simulink model "smlnk_hw4"  (R2019b)
settings: Solver=VariableStepAuto  StartTime=0.0  StopTime=15  RelTol=1e-3
undefined symbols (not defined in the file): C, m, sys, x0
settings Model: Creator=maximemeurisse  LastModifiedBy=maximemeurisse

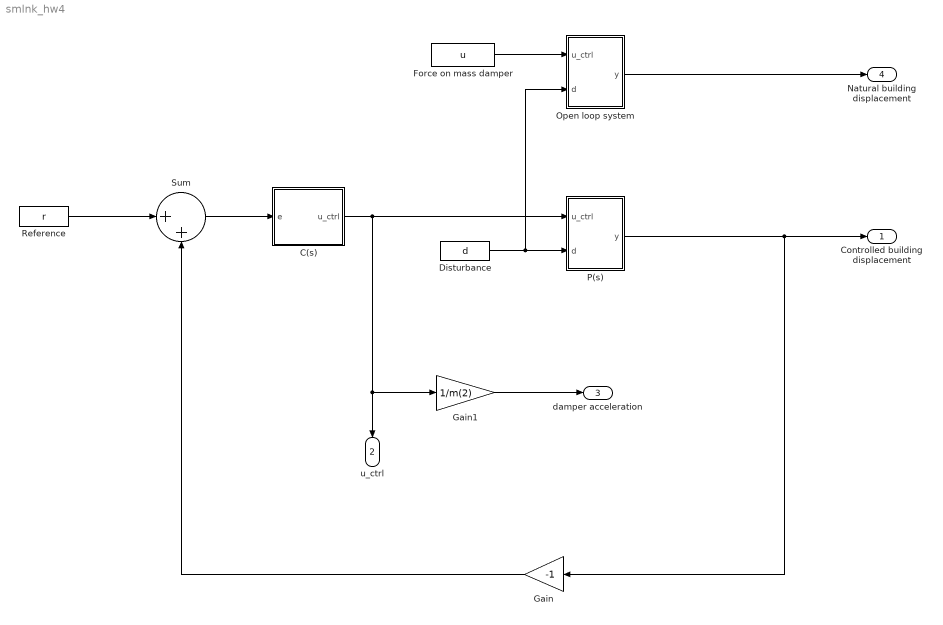
== system smlnk_hw4 ==
  C(s) : Subsystem
  Disturbance : FromWorkspace  VariableName=d  SampleTime=0
  Force on mass damper : FromWorkspace  VariableName=u  SampleTime=0
  Gain : Gain  Gain=-1
  Gain1 : Gain  Gain=1/m(2)
  Open loop system : Subsystem
  P(s) : Subsystem
  Reference : FromWorkspace  VariableName=r  SampleTime=0
  Sum : Sum  Inputs=|++
  Controlled building displacement : Outport
  u_ctrl : Outport  Port=2
  damper acceleration : Outport  Port=3
  Natural building displacement : Outport  Port=4
  wires:
  Gain/1 -> Sum/2
  Sum/1 -> C(s)/1(e)
  Reference/1 -> Sum/1
  Gain1/1 -> damper acceleration/1
  C(s)/1(u_ctrl) -> P(s)/1(u_ctrl), u_ctrl/1, Gain1/1
  P(s)/1(y) -> Gain/1, Controlled building displacement/1
  Disturbance/1 -> Open loop system/2(d), P(s)/2(d)
  Open loop system/1(y) -> Natural building displacement/1
  Force on mass damper/1 -> Open loop system/1(u_ctrl)

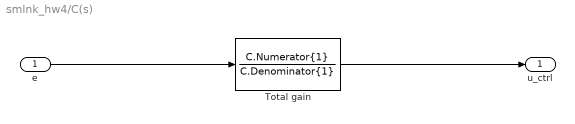
== system smlnk_hw4/C(s) ==
  e : Inport
  Total gain : TransferFcn  Numerator=C.Numerator{1}  Denominator=C.Denominator{1}
  u_ctrl : Outport
  wires:
  e/1 -> Total gain/1
  Total gain/1 -> u_ctrl/1

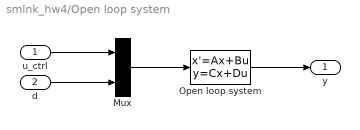
== system smlnk_hw4/Open loop system ==
  u_ctrl : Inport
  d : Inport  Port=2
  Mux : Mux  Inputs=2
  Open loop system : StateSpace  A=sys.A  B=sys.B  C=sys.C  D=sys.D  InitialCondition=x0
  y : Outport
  wires:
  d/1 -> Mux/2
  u_ctrl/1 -> Mux/1
  Open loop system/1 -> y/1
  Mux/1 -> Open loop system/1

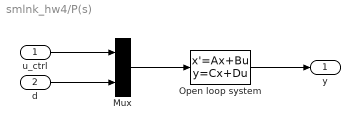
== system smlnk_hw4/P(s) ==
  u_ctrl : Inport
  d : Inport  Port=2
  Mux : Mux  Inputs=2
  Open loop system : StateSpace  A=sys.A  B=sys.B  C=sys.C  D=sys.D  InitialCondition=x0
  y : Outport
  wires:
  d/1 -> Mux/2
  u_ctrl/1 -> Mux/1
  Open loop system/1 -> y/1
  Mux/1 -> Open loop system/1
